simulink model "Clutchless_P2_Parallel_ETE"  (R2017b)
settings: Solver=FixedStepAuto  StartTime=0.0  StopTime=length(Speed)  FixedStep=0.01  MaxStep=0.01  RelTol=1e-3  EnableMultiTasking=on
PostLoadFcn:
  | , if any(exist('dsrtsu_mdlpostloadfcn', 'file') == [2, 3, 6]), try dsrtsu_mdlpostloadfcn('Execute', bdroot); catch fprintf('Error in PostLoadFcn (dsrtsu_mdlpostloadfcn) for model "%s":\n %s\n', bdroot, lasterr); end, end,
undefined symbols (not defined in the file): ABSEnable, Actuators, air, APP1_OOR, APP2_OOR, APP_Mismatch, Brk_Flt, cal, ClutchEngag, Clutchless_HSC_ETE, CS_On_Control, Driver, eng, Engine, EngOverTemp, ENGTRQ_MSMCH_Degraded_CP, ENGTRQ_MSMCH_ErrCritical_CP, ENGTRQ_MSMCH_LimpHome_CP, EngTrqMismatch, env, ess, ESSOverTemp, gb, KeyPos_Flt, KeyPosition, lib_Actuators, lib_Clutchless_HSC_ETE, lib_Driver, lib_EMachine_2017a, lib_Sensors_2017a, LossCAN, Machine, max_vehicle_rad_air_flow, MCUOverTemp, mot, MotDirMismatch, MotOverTemp, MotTrqMismatch, mph2ms, PRNDL_Flt, RegenBrkDisable, RegenFault, Sensors, ShiftLeverPosition, Speed, SW_CS_ON, SW_Engine_ON, t_amb, time, tloop
libraries: simulink x97, Pneumatic_lib x11, nesl_utility x9, EC2_libraries x7, powerlib_meascontrol x2, CalculationGallon x1, lib_Chassis x1, lib_DCDC x1, lib_Differential x1, lib_HVESS x1, fl_lib x1, lib_OBC x1
(part 4 of 9)

== system Clutchless_P2_Parallel_ETE/Camaro Plant Model/E-Machine/IMG Plant2/Motor_Plant/Efficiency Calcs ==
  Speed_rpm : Inport
  Torq_cmd_Nm : Inport  Port=2
  Batt_volt : Inport  Port=3
  Abs1 : Abs
  Constant : Constant
  Constant1 : Constant  Value=0
  Current_consum : Product  Inputs=*/
  Efficiency Map : Lookup_n-D  BreakpointsForDimension1=mot.map.trqindex  BreakpointsForDimension2=mot.map.spdindex  Table=mot.map.eff  InternalRulePriority=Speed  RndMeth=Simplest  InputSameDT=on
  Electrical power motoring : Product  Inputs=*//
  Electrical power regen : Product  Inputs=***
  Gain : Gain  Gain=2*3.14/60
  Gain1 : Gain  Gain=-1
  MCU_eff : Constant  Value=0.97
  Mech_power : Product  Inputs=**
  MinMax : MinMax  Function=max  Inputs=2
  MinMax1 : MinMax  Function=max  Inputs=2
  Saturation : Saturate  UpperLimit=400  LowerLimit=-400
  Switch : Switch  Criteria=u2 > Threshold
  Switch1 : Switch  Criteria=u2 > Threshold  Threshold=100
  min_eff : Constant  Value=0.1
  Mot_current : Outport
  Mech_power_W : Outport  Port=2
  Elec_power_W : Outport  Port=3
  wires:
  Constant1/1 -> Switch1/3
  Switch/1 -> Switch1/1  "Elec_power_W"
  Gain1/1 -> Saturation/1  "Mot_current_A"
  Constant/1 -> MinMax1/2
  MinMax1/1 -> Current_consum/2
  Efficiency Map/1 -> MinMax/1
  Switch1/1 -> Current_consum/1, Elec_power_W/1  "Elec_power_W"
  min_eff/1 -> MinMax/2
  Electrical power motoring/1 -> Switch/1
  MCU_eff/1 -> Electrical power motoring/3, Electrical power regen/3
  Mech_power/1 -> Mech_power_W/1, Electrical power regen/1, Electrical power motoring/1  "Mech_power_W"
  Abs1/1 -> Efficiency Map/1
  Batt_volt/1 -> MinMax1/1, Switch1/2
  Gain/1 -> Mech_power/1
  Saturation/1 -> Mot_current/1  "Mot_current_A"
  Current_consum/1 -> Gain1/1
  MinMax/1 -> Electrical power regen/2, Electrical power motoring/2
  Electrical power regen/1 -> Switch/3
  Torq_cmd_Nm/1 -> Switch/2, Abs1/1, Mech_power/2
  Speed_rpm/1 -> Gain/1, Efficiency Map/2

== system Clutchless_P2_Parallel_ETE/Camaro Plant Model/E-Machine/IMG Plant2/Thermal/Motor Thermal ==
  In1 : Inport
  Add1 : Sum  Inputs=+-
  Add2 : Sum
  Divide : Product  Inputs=*/
  Lower Limit : Subsystem  mask{Lolimit=t_amb+20}
      mask prompts: Lolimit "Lower Limit"
  Memory1 : Memory
  Motor Mass : Constant  Value=mot.plant.init.motor_mass
  Product : Product  RndMeth=Zero
  "Pump " : Constant  Value=0
  Specific Heat Cap Aluminum : Constant  Value=mot.plant.init.specific_heat
  tloop : Gain  Gain=tloop
  Out1 : Outport
  wires:
  Add1/1 -> tloop/1
  In1/1 -> Add1/1
  "Pump "/1 -> Add1/2
  Motor Mass/1 -> Product/1  "kg"
  tloop/1 -> Divide/1  "J"
  Divide/1 -> Add2/1
  Lower Limit/1(Out1) -> Memory1/1, Out1/1
  Add2/1 -> Lower Limit/1(In1)
  Memory1/1 -> Add2/2
  Product/1 -> Divide/2
  Specific Heat Cap Aluminum/1 -> Product/2  "J/kg*K"

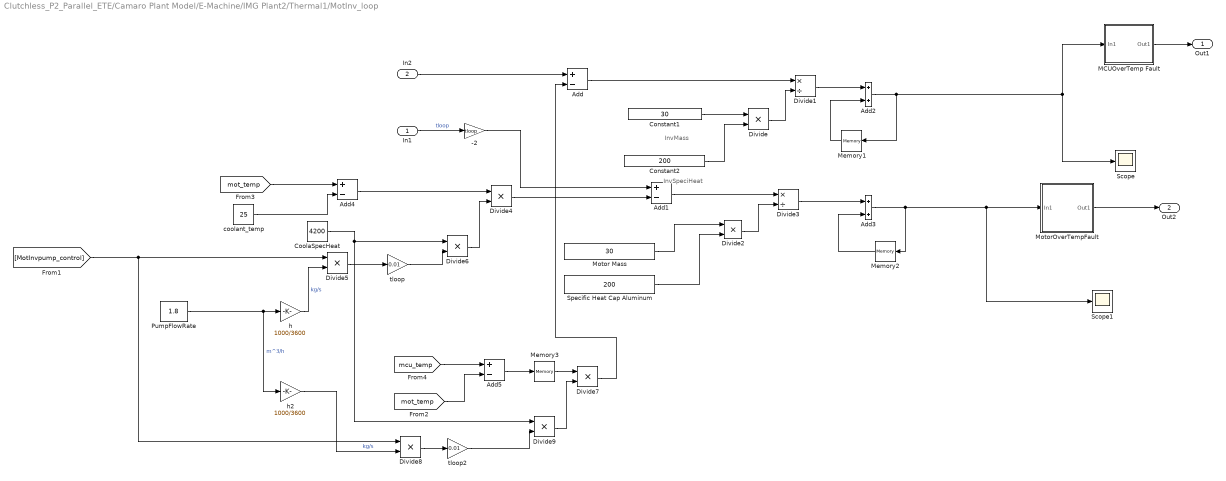
== system Clutchless_P2_Parallel_ETE/Camaro Plant Model/E-Machine/IMG Plant2/Thermal1/MotInv_loop ==
  note: InvMass
  note: InvSpeciHeat
  In1 : Inport
  In2 : Inport  Port=2
  -2 : Gain  Gain=tloop
  Add{,1,4..5} (4 alike) : Sum  Inputs=+-
  Add2 : Sum
  Add3 : Sum
  Constant1 : Constant  Value=30
  Constant2 : Constant  Value=200
  CoolaSpecHeat : Constant  Value=4200
  Divide{,2,4..9} (8 alike) : Product  Inputs=**
  Divide1 : Product  Inputs=*/
  Divide3 : Product  Inputs=*/
  MCUOverTemp Fault : Subsystem
  Memory1 : Memory  InitialCondition=25
  Memory2 : Memory  InitialCondition=25
  Memory3 : Memory
  Motor Mass : Constant  Value=30
  MotorOverTempFault : Subsystem
  PumpFlowRate : Constant  Value=1.8
  Scope : Scope
  Scope1 : Scope
  Specific Heat Cap Aluminum : Constant  Value=200
  coolant_temp : Constant  Value=25
  h : Gain  Gain=1000/3600
  h2 : Gain  Gain=1000/3600
  tloop : Gain  Gain=0.01
  tloop2 : Gain  Gain=0.01
  Out1 : Outport
  Out2 : Outport  Port=2
  wires:
  [MotInvpump_control] -> Divide5/1, Divide8/1
  -2/1 -> Add1/1
  In2/1 -> Add/1
  In1/1 -> -2/1  "tloop"
  [mot_temp] -> Add5/2
  [mcu_temp] -> Add5/1
  [mot_temp] -> Add4/1
  MotorOverTempFault/1(Out1) -> Out2/1
  MCUOverTemp Fault/1(Out1) -> Out1/1
  Memory3/1 -> Divide7/1
  Add5/1 -> Memory3/1
  Divide4/1 -> Add1/2
  tloop2/1 -> Divide9/2
  Divide8/1 -> tloop2/1
  Divide9/1 -> Divide7/2
  h2/1 -> Divide8/2  "kg/s"
  PumpFlowRate/1 -> h/1, h2/1  "m^3/h"
  CoolaSpecHeat/1 -> Divide9/1, Divide6/1
  tloop/1 -> Divide6/2
  h/1 -> Divide5/2  "kg/s"
  Divide7/1 -> Add/2
  Divide1/1 -> Add2/1
  Motor Mass/1 -> Divide2/1
  Constant2/1 -> Divide/2
  Divide2/1 -> Divide3/2
  Add2/1 -> Memory1/1, Scope/1, MCUOverTemp Fault/1(In1)
  Divide5/1 -> tloop/1
  Divide3/1 -> Add3/1
  Divide6/1 -> Divide4/2
  Add3/1 -> Memory2/1, MotorOverTempFault/1(In1), Scope1/1
  Add4/1 -> Divide4/1
  Memory2/1 -> Add3/2
  Add/1 -> Divide1/1
  Constant1/1 -> Divide/1
  Specific Heat Cap Aluminum/1 -> Divide2/2
  Divide/1 -> Divide1/2
  coolant_temp/1 -> Add4/2
  Memory1/1 -> Add2/2
  Add1/1 -> Divide3/1

== system Clutchless_P2_Parallel_ETE/Camaro Plant Model/E-Machine/IMG Plant2/Thermal1/Motor Thermal ==
  In1 : Inport
  Add1 : Sum  Inputs=+-
  Add2 : Sum
  Divide : Product  Inputs=*/
  Lower Limit : Subsystem  mask{Lolimit=t_amb+20}
      mask prompts: Lolimit "Lower Limit"
  Memory1 : Memory
  Motor Mass : Constant  Value=mot.plant.init.motor_mass
  Product : Product  RndMeth=Zero
  "Pump " : Constant  Value=0
  Specific Heat Cap Aluminum : Constant  Value=mot.plant.init.specific_heat
  tloop : Gain  Gain=tloop
  Out1 : Outport
  wires:
  Add1/1 -> tloop/1
  In1/1 -> Add1/1
  "Pump "/1 -> Add1/2
  Motor Mass/1 -> Product/1  "kg"
  tloop/1 -> Divide/1  "J"
  Divide/1 -> Add2/1
  Lower Limit/1(Out1) -> Memory1/1, Out1/1
  Add2/1 -> Lower Limit/1(In1)
  Memory1/1 -> Add2/2
  Product/1 -> Divide/2
  Specific Heat Cap Aluminum/1 -> Product/2  "J/kg*K"

== system Clutchless_P2_Parallel_ETE/Camaro Plant Model/E-Machine/IMG Plant2/Torque Calculation/electric machine filter ==
  trq : Inport
  Interval Test : simulink/Logic and Bit Operations/Interval Test  IntervalClosedRight=on  uplimit=0.5  IntervalClosedLeft=on  lowlimit=-0.5  OutDataTypeStr=boolean
  Switch : Switch  Threshold=0.5
  electric machine time response : TransferFcn  Denominator=[mot.plant.init.time_response 1]
  filtered : Outport
  wires:
  Switch/1 -> filtered/1
  trq/1 -> Switch/1, electric machine time response/1, Interval Test/1
  Interval Test/1 -> Switch/2
  electric machine time response/1 -> Switch/3

== system Clutchless_P2_Parallel_ETE/Camaro Plant Model/E-Machine/IMG Plant2/Torque Calculation/max torque  ==
  cmd : Inport
  speed : Inport  Port=2
  Memory : Memory
  Peak trq max - Motoring : Lookup  InputValues=mot.plant.init.regen.trq_max.idx1_spd  Table=mot.plant.init.motor.trq_max.map  LookUpMeth=Interpolation-Use End Values  SaturateOnIntegerOverflow=on
  Peak trq max - Regen : Lookup  InputValues=mot.plant.init.regen.trq_max.idx1_spd  Table=mot.plant.init.regen.trq_max.map  LookUpMeth=Interpolation-Use End Values  SaturateOnIntegerOverflow=on
  Switch1 : Switch  SaturateOnIntegerOverflow=on
  rad/s  to RPM : Gain  Gain=30/pi
  max torque : Outport
  wires:
  Peak trq max - Regen/1 -> Switch1/3
  rad/s  to RPM/1 -> Memory/1
  Memory/1 -> Peak trq max - Regen/1, Peak trq max - Motoring/1
  Switch1/1 -> max torque/1
  cmd/1 -> Switch1/2
  speed/1 -> rad/s  to RPM/1
  Peak trq max - Motoring/1 -> Switch1/1

== system Clutchless_P2_Parallel_ETE/Camaro Plant Model/E-Machine/Soft MCU/Subsystem/MCU_RollingAliveCnt ==
  Counter Free-Running : simulink/Sources/Counter Free-Running  NumBits=4  tsamp=-1
  Out1 : Outport
  wires:
  Counter Free-Running/1 -> Out1/1  "MCURollingAliveCnt [0 1 2 3]"

== system Clutchless_P2_Parallel_ETE/Camaro Plant Model/E-Machine/Soft MCU/Torque Calculation1/max torque  ==
  Req : Inport
  speed : Inport  Port=2
  torque : Inport  Port=3
  2-D Lookup Table : Lookup_n-D  Commented=on  BreakpointsForDimension1=mot.plant.init.eff_trq.idx2_trq  BreakpointsForDimension2=mot.plant.init.eff_trq.idx1_spd  Table=mot.plant.init.eff_trq.map  InternalRulePriority=Speed  RndMeth=Simplest  InputSameDT=on
  Abs : Abs  SaturateOnIntegerOverflow=on
  Abs1 : Abs  Commented=on
  Abs2 : Abs  Commented=on
  Constant : Constant  Commented=on  Value=84500
  Cont trq max - Motoring : Lookup  InputValues=mot.plant.init.motor.trq_cont.idx1_spd  Table=mot.plant.init.motor.trq_cont.map  LookUpMeth=Interpolation-Use End Values  SaturateOnIntegerOverflow=on
  Cont trq max - Regen : Lookup  InputValues=mot.plant.init.regen.trq_cont.idx1_spd  Table=mot.plant.init.regen.trq_cont.map  LookUpMeth=Interpolation-Use End Values  SaturateOnIntegerOverflow=on
  Divide : Product  Commented=on  Inputs=**/
  Divide by zero : Subsystem  Commented=on
  Gain2 : Gain  Commented=on  Gain=1/100
  Heat index : Subsystem
  Memory : Memory
  Peak trq max - Motoring : Lookup  Commented=on  InputValues=mot.plant.init.regen.trq_max.idx1_spd  Table=mot.plant.init.motor.trq_max.map  LookUpMeth=Interpolation-Use End Values  SaturateOnIntegerOverflow=on
  Peak trq max - Motoring1 : Lookup  InputValues=mot.plant.init.regen.trq_max.idx1_spd  Table=mot.plant.init.motor.trq_max.map  LookUpMeth=Interpolation-Use End Values  SaturateOnIntegerOverflow=on
  Peak trq max - Regen : Lookup  InputValues=mot.plant.init.regen.trq_max.idx1_spd  Table=mot.plant.init.regen.trq_max.map  LookUpMeth=Interpolation-Use End Values  SaturateOnIntegerOverflow=on
  Product2 : Product  SaturateOnIntegerOverflow=on  InputSameDT=on  OutDataTypeStr=Inherit: Same as first input
  Product3 : Product  SaturateOnIntegerOverflow=on  InputSameDT=on  OutDataTypeStr=Inherit: Same as first input
  Product5 : Product  SaturateOnIntegerOverflow=on  InputSameDT=on  OutDataTypeStr=Inherit: Same as first input
  RPM to rad/s : Gain  Commented=on  Gain=pi/30
  Sign : Signum
  Sum : Sum  SaturateOnIntegerOverflow=on  InputSameDT=on  OutDataTypeStr=Inherit: Same as first input
  Sum1 : Sum  Inputs=-+  SaturateOnIntegerOverflow=on  InputSameDT=on  OutDataTypeStr=Inherit: Same as first input
  Switch : Switch  SaturateOnIntegerOverflow=on
  Switch1 : Switch  SaturateOnIntegerOverflow=on
  cst : Constant
  max torque : Outport
  wires:
  Heat index/1(Heat index) -> Product2/2, Sum1/1
  cst/1 -> Sum1/2
  Product3/1 -> Sum/2
  Sum1/1 -> Product3/1
  Product2/1 -> Sum/1
  Switch1/1 -> Product3/2
  Switch/1 -> Heat index/1(cont torque), Product2/1
  Peak trq max - Regen/1 -> Switch1/3
  Cont trq max - Regen/1 -> Switch/3
  Cont trq max - Motoring/1 -> Switch/1
  torque/1 -> Heat index/2(torque)
  Abs/1 -> Product5/2
  Sum/1 -> Abs/1, Sign/1
  Product5/1 -> max torque/1
  Sign/1 -> Product5/1
  Memory/1 -> Cont trq max - Motoring/1, Cont trq max - Regen/1, Peak trq max - Motoring1/1, Peak trq max - Regen/1
  speed/1 -> Memory/1
  Constant/1 -> Divide/1
  RPM to rad/s/1 -> Divide by zero/1(In1)
  Abs2/1 -> 2-D Lookup Table/2
  Abs1/1 -> 2-D Lookup Table/1
  2-D Lookup Table/1 -> Gain2/1
  Gain2/1 -> Divide/2
  Req/1 -> Switch/2, Switch1/2
  Divide by zero/1(Out1) -> Divide/3
  Peak trq max - Motoring1/1 -> Switch1/1

== system Clutchless_P2_Parallel_ETE/Camaro Plant Model/E-Machine/Soft MCU/Torque Calculation2/max torque  ==
  Req : Inport
  speed : Inport  Port=2
  torque : Inport  Port=3
  2-D Lookup Table : Lookup_n-D  Commented=on  BreakpointsForDimension1=mot.plant.init.eff_trq.idx2_trq  BreakpointsForDimension2=mot.plant.init.eff_trq.idx1_spd  Table=mot.plant.init.eff_trq.map  InternalRulePriority=Speed  RndMeth=Simplest  InputSameDT=on
  Abs : Abs  SaturateOnIntegerOverflow=on
  Abs1 : Abs  Commented=on
  Abs2 : Abs  Commented=on
  Constant : Constant  Commented=on  Value=84500
  Cont trq max - Motoring : Lookup  InputValues=mot.plant.init.motor.trq_cont.idx1_spd  Table=mot.plant.init.motor.trq_cont.map  LookUpMeth=Interpolation-Use End Values  SaturateOnIntegerOverflow=on
  Cont trq max - Regen : Lookup  InputValues=mot.plant.init.regen.trq_cont.idx1_spd  Table=mot.plant.init.regen.trq_cont.map  LookUpMeth=Interpolation-Use End Values  SaturateOnIntegerOverflow=on
  Divide : Product  Commented=on  Inputs=**/
  Divide by zero : Subsystem  Commented=on
  Gain2 : Gain  Commented=on  Gain=1/100
  Heat index : Subsystem
  Memory : Memory
  Peak trq max - Motoring : Lookup  Commented=on  InputValues=mot.plant.init.regen.trq_max.idx1_spd  Table=mot.plant.init.motor.trq_max.map  LookUpMeth=Interpolation-Use End Values  SaturateOnIntegerOverflow=on
  Peak trq max - Motoring1 : Lookup  InputValues=mot.plant.init.regen.trq_max.idx1_spd  Table=mot.plant.init.motor.trq_max.map  LookUpMeth=Interpolation-Use End Values  SaturateOnIntegerOverflow=on
  Peak trq max - Regen : Lookup  InputValues=mot.plant.init.regen.trq_max.idx1_spd  Table=mot.plant.init.regen.trq_max.map  LookUpMeth=Interpolation-Use End Values  SaturateOnIntegerOverflow=on
  Product2 : Product  SaturateOnIntegerOverflow=on  InputSameDT=on  OutDataTypeStr=Inherit: Same as first input
  Product3 : Product  SaturateOnIntegerOverflow=on  InputSameDT=on  OutDataTypeStr=Inherit: Same as first input
  Product5 : Product  SaturateOnIntegerOverflow=on  InputSameDT=on  OutDataTypeStr=Inherit: Same as first input
  RPM to rad/s : Gain  Commented=on  Gain=pi/30
  Sign : Signum
  Sum : Sum  SaturateOnIntegerOverflow=on  InputSameDT=on  OutDataTypeStr=Inherit: Same as first input
  Sum1 : Sum  Inputs=-+  SaturateOnIntegerOverflow=on  InputSameDT=on  OutDataTypeStr=Inherit: Same as first input
  Switch : Switch  SaturateOnIntegerOverflow=on
  Switch1 : Switch  SaturateOnIntegerOverflow=on
  cst : Constant
  max torque : Outport
  wires:
  Heat index/1(Heat index) -> Product2/2, Sum1/1
  cst/1 -> Sum1/2
  Product3/1 -> Sum/2
  Sum1/1 -> Product3/1
  Product2/1 -> Sum/1
  Switch1/1 -> Product3/2
  Switch/1 -> Heat index/1(cont torque), Product2/1
  Peak trq max - Regen/1 -> Switch1/3
  Cont trq max - Regen/1 -> Switch/3
  Cont trq max - Motoring/1 -> Switch/1
  torque/1 -> Heat index/2(torque)
  Abs/1 -> Product5/2
  Sum/1 -> Abs/1, Sign/1
  Product5/1 -> max torque/1
  Sign/1 -> Product5/1
  Memory/1 -> Cont trq max - Motoring/1, Cont trq max - Regen/1, Peak trq max - Motoring1/1, Peak trq max - Regen/1
  speed/1 -> Memory/1
  Constant/1 -> Divide/1
  RPM to rad/s/1 -> Divide by zero/1(In1)
  Abs2/1 -> 2-D Lookup Table/2
  Abs1/1 -> 2-D Lookup Table/1
  2-D Lookup Table/1 -> Gain2/1
  Gain2/1 -> Divide/2
  Req/1 -> Switch/2, Switch1/2
  Divide by zero/1(Out1) -> Divide/3
  Peak trq max - Motoring1/1 -> Switch1/1

== system Clutchless_P2_Parallel_ETE/Camaro Plant Model/ICE Simple1/Engine Plant Modified/Core Engine/Core Engine1 ==
  Engine Speed (RPM) : Inport
  CO : Lookup2D  RowIndex=Engine.Engine.Emissions.SPEED  ColumnIndex=Engine.Engine.Emissions.TQ  Table=Engine.Engine.Emissions.CO/1000  LookUpMeth=Interpolation-Use End Values
  CO2 : Lookup2D  RowIndex=Engine.Engine.Emissions.SPEED  ColumnIndex=Engine.Engine.Emissions.TQ  Table=Engine.Engine.Emissions.CO2/1000  LookUpMeth=Interpolation-Use End Values
  Controlled Pneumatic Flow Rate Source : Pneumatic_lib/Pneumatic Sources/Controlled Pneumatic Flow Rate Source
  Fuel Flow : Lookup2D  RowIndex=Engine.Engine.FuelFlow.SPEED  ColumnIndex=Engine.Engine.FuelFlow.TQ  Table=Engine.Engine.FuelFlow.FuelFlow  LookUpMeth=Interpolation-Use End Values
  HC : Lookup2D  RowIndex=Engine.Engine.Emissions.SPEED  ColumnIndex=Engine.Engine.Emissions.TQ  Table=Engine.Engine.Emissions.HC/1000  LookUpMeth=Interpolation-Use End Values
  Half of Displacement : Gain  Gain=Engine.DisplacedVolume/(2*1000)
  Ideal Gas Constant R : Gain  Gain=287
  Kg/s to g/s : Gain  Gain=1000
  LP Filter1 : TransferFcn  Denominator=[0.001 1]
  Memory : Memory
  NOx : Lookup2D  RowIndex=Engine.Engine.Emissions.SPEED  ColumnIndex=Engine.Engine.Emissions.TQ  Table=Engine.Engine.Emissions.NOx/1000  LookUpMeth=Interpolation-Use End Values
  Power Enrichment Torque Boundary vs Speed : Lookup_n-D  NumberOfTableDimensions=1  BreakpointsForDimension1=Engine.Engine.PEBound.SPEED  Table=Engine.Engine.PEBound.PEBound  ExtrapMethod=Clip  InternalRulePriority=Speed  RndMeth=Simplest  InputSameDT=on
  Product : Product  Inputs=***
  RPM to RPS : Gain  Gain=1/60
  Relational Operator : RelationalOperator  Operator=>  OutDataTypeStr=boolean  RndMeth=Nearest
  Simulink-PS Converter2 : nesl_utility/Simulink-PS Converter  PhysicalDomain=network_engine_domain  SubClassName=ps_input  LeftPortType=input  RightPortType=output  PseudoPeriodic=off  Frequencies=[]  NoiseDistribution=none  NoiseParameters=[]  Unit=kg/s  AffineConversion=off  FilteringAndDerivatives=zero  SimscapeFilterOrder=1  InputFilterTimeConstant=.001  UdotUserProvided=0
  Speed-Density Mass Flow : Product  Inputs=*/
  Torque : Lookup2D  RowIndex=Engine.Engine.TQ.SPEED  ColumnIndex=Engine.Engine.TQ.MAF  Table=Engine.Engine.TQ.TQ  LookUpMeth=Interpolation-Use End Values
  Upstream States : Subsystem
  Volumetric Efficiency : Lookup2D  RowIndex=Engine.Engine.VE.MAP  ColumnIndex=Engine.Engine.VE.SPEED  Table=Engine.Engine.VE.VE  LookUpMeth=Interpolation-Use End Values
  A : PMIOPort  Port=1  Side=Left
  B : PMIOPort  Port=2  Side=Right
  Brake Torque (Nm) : Outport
  Fuel Flow (g/s) : Outport  Port=2
  PE Status : Outport  Port=3
  HC (g/s) : Outport  Port=4
  CO (g/s) : Outport  Port=5
  NOx (g/s) : Outport  Port=6
  CO2 (g/s) : Outport  Port=7
  Intake Port Airflow (g/s) : Outport  Port=8
  wires:
  Upstream States/1(P (Pa)) -> Volumetric Efficiency/1, Product/3
  Volumetric Efficiency/1 -> Product/1
  Ideal Gas Constant R/1 -> Speed-Density Mass Flow/2
  Product/1 -> Speed-Density Mass Flow/1
  Upstream States/2(T (K)) -> Ideal Gas Constant R/1
  RPM to RPS/1 -> Half of Displacement/1
  Half of Displacement/1 -> Product/2
  Kg/s to g/s/1 -> [INTAKEPORTFLOW]
  Torque/1 -> Brake Torque (Nm)/1, Relational Operator/1, Memory/1  "Brake Torque"
  [INTAKEPORTFLOW] -> Torque/2
  Fuel Flow/1 -> Fuel Flow (g/s)/1  "Fuel Flow"
  Engine Speed (RPM)/1 -> Torque/1, Fuel Flow/1, HC/1, CO/1, NOx/1, Power Enrichment Torque Boundary vs Speed/1, CO2/1, Volumetric Efficiency/2, RPM to RPS/1
  Memory/1 -> CO2/2, NOx/2, CO/2, HC/2, Fuel Flow/2
  Power Enrichment Torque Boundary vs Speed/1 -> Relational Operator/2
  Relational Operator/1 -> PE Status/1
  HC/1 -> HC (g/s)/1
  CO/1 -> CO (g/s)/1
  NOx/1 -> NOx (g/s)/1
  CO2/1 -> CO2 (g/s)/1
  [INTAKEPORTFLOW] -> Intake Port Airflow (g/s)/1
  Speed-Density Mass Flow/1 -> LP Filter1/1, Kg/s to g/s/1
  LP Filter1/1 -> Simulink-PS Converter2/1
  connections:
  A/RConn1 -- Controlled Pneumatic Flow Rate Source/RConn1 -- Upstream States/LConn1
  Simulink-PS Converter2/RConn1 -- Controlled Pneumatic Flow Rate Source/RConn2
  B/RConn1 -- Controlled Pneumatic Flow Rate Source/LConn1

== system Clutchless_P2_Parallel_ETE/Camaro Plant Model/ICE Simple1/Engine Plant Modified/Core Engine/Crank Process/function ==
  EngSpd : Inport
  f : TriggerPort  TriggerType=function-call  VariantControl=Variant
      settings: CopyFcn=Stateflow.SLINSF.SimulinkMan.removeBlockPreDeleteFcn  PreDeleteFcn=Stateflow.SLINSF.SimulinkMan.unsafePredeleteFcn
  1-D Lookup Table : Lookup_n-D  NumberOfTableDimensions=1  BreakpointsForDimension1=[0 50 120 210 300 320 340 350 400]  Table="[90 90 90 10 5 5  5 5 5]"  InternalRulePriority=Speed  RndMeth=Simplest  InputSameDT=on
  CrankTrq : Outport
  wires:
  EngSpd/1 -> 1-D Lookup Table/1
  1-D Lookup Table/1 -> CrankTrq/1

== system Clutchless_P2_Parallel_ETE/Camaro Plant Model/ICE Simple1/Engine Plant Modified/Core Engine/EngEfficiency1 ==
  note: Mechanical Power [W]
  Torque : Inport
  Speed : Inport  Port=2
  Fuel Consumption : Inport  Port=3
  Divide by Zero Fix : Subsystem
  Divide_by_Zero_Fix1 : EC2_libraries/Divide_by_Zero_Fix  Commented=on
  From1 : From  Commented=on  GotoTag=Wh_out
  From2 : From  Commented=on  GotoTag=Wh_in
  Goto1 : Goto  Commented=on  GotoTag=Wh_out
  Goto2 : Goto  Commented=on  GotoTag=Wh_in
  Integrator1 : Integrator  Commented=on  LimitOutput=on  LowerSaturationLimit=0
  Integrator2 : Integrator  Commented=on  LimitOutput=on  LowerSaturationLimit=0
  OnlyPositiveEnergy : Saturate  Commented=on  UpperLimit=inf  LowerLimit=0
  Percentage Efficiency : Gain  Gain=100
  Product : Product  RndMeth=Zero
  "RPM to rad/s " : Gain  Gain=pi/30
  Scope : Scope  NumInputPorts=2
  Specific Energy LHV in J/kg : Gain  Gain=Engine.Fuel.Lower_Heating_Value/1000
  Sum : Sum  Inputs=-+
  To Workspace7 : ToWorkspace  Commented=on  VariableName=eng_Wh_pos_eff_hist  SampleTime=-1
      settings: Decimation=WORKSPACE_DECIMATION
  engine_efficiency : Scope
  limit_efficiency[0-100%] : Saturate  UpperLimit=100  LowerLimit=0
  PowerLoss : Outport
  wires:
  limit_efficiency[0-100%]/1 -> engine_efficiency/1
  Sum/1 -> PowerLoss/1  "Losses [W]"
  Fuel Consumption/1 -> Specific Energy LHV in J/kg/1
  Specific Energy LHV in J/kg/1 -> Divide by Zero Fix/2(Divide), Sum/2, Integrator2/1, Scope/2  "Thermal Power [W]"
  Torque/1 -> Product/2  "Nm"
  Speed/1 -> "RPM to rad/s "/1  "rpm"
  Percentage Efficiency/1 -> limit_efficiency[0-100%]/1  "Efficiency [%]"
  Divide by Zero Fix/1(Output) -> Percentage Efficiency/1
  Product/1 -> Scope/1, Divide by Zero Fix/1(Multiply), OnlyPositiveEnergy/1, Sum/1  "wer [W]"
  Divide_by_Zero_Fix1/1 -> To Workspace7/1
  From1/1 -> Divide_by_Zero_Fix1/1
  From2/1 -> Divide_by_Zero_Fix1/2
  Integrator1/1 -> Goto1/1
  OnlyPositiveEnergy/1 -> Integrator1/1
  Integrator2/1 -> Goto2/1
  "RPM to rad/s "/1 -> Product/1

== system Clutchless_P2_Parallel_ETE/Camaro Plant Model/ICE Simple1/Engine Plant Modified/Core Engine/EngineThermal1 ==
  note: Temp Delta C deg
  PowerLoss : Inport
  Divide : Product  Inputs=*/
  Divide1 : Product  Inputs=**
  Engine Mass : Constant  Value=Engine.Mass
  Memory : Memory  InitialCondition=Engine.Init_T_amb
  Memory1 : Memory
  Product : Product  RndMeth=Zero
  Specific Heat Cap Aluminum : Constant  Value=Engine.Specific_Heat
  Sum : Sum  Inputs=|++
  Sum1 : Sum  Inputs=|+-
  Terminator : Terminator
  tloop : Constant  Value=0.01
  Temp[degC] : Outport
  tag scope: Heat_Transfer_Eng=global
  wires:
  Memory1/1 -> Sum1/2
  Divide1/1 -> Divide/1  "J"
  Sum1/1 -> Divide1/2
  Memory/1 -> Sum/2
  PowerLoss/1 -> Sum1/1, [Heat_Transfer_Eng]  "J/s"
  Engine Mass/1 -> Product/1  "kg"
  Specific Heat Cap Aluminum/1 -> Product/2  "J/kg*K"
  Product/1 -> Divide/2
  Sum/1 -> Memory/1, Temp[degC]/1
  Divide/1 -> Sum/1
  tloop/1 -> Divide1/1
  [Heat_Reject_Eng] -> Memory1/1
  [Heat_Transfer_Eng] -> Terminator/1

== system Clutchless_P2_Parallel_ETE/Camaro Plant Model/ICE Simple1/Engine Plant Modified/Core Engine/Intake Manifold1 ==
  Heat-Transfer Neglected : fl_lib/Thermal/Thermal Elements/Perfect Insulator  T_specify=off  T_priority=None  T=0 K  T_nominal_specify=off  T_nominal_unit=K  T_nominal_value=1
      settings: SourceProductName=Simscape
  Intake Manifold Volume1 : Pneumatic_lib/Pneumatic Elements/Constant Volume Pneumatic Chamber  Volume=Engine.IntakeManifold.Volume l  pressure_specify=on  pressure_priority=High  pressure=26 kPa  pressure_nominal_specify=off  pressure_nominal_unit=Pa  pressure_nominal_value=1  temperature_specify=on  temperature_priority=High  temperature=20 K  temperature_nominal_specify=off  temperature_nominal_unit=K  temperature_nominal_value=1  gas_flow_specify=off  gas_flow_priority=High  gas_flow=0 kg/s  gas_flow_nominal_specify=off  gas_flow_nominal_unit=kg/s  gas_flow_nominal_value=1  heat_flow_specify=off  heat_flow_priority=High  heat_flow=0 J/s  heat_flow_nominal_specify=off  heat_flow_nominal_unit=J/s  heat_flow_nominal_value=1  heat_exch_flow_specify=off  heat_exch_flow_priority=High  heat_exch_flow=0 J/s  heat_exch_flow_nominal_specify=off  heat_exch_flow_nominal_unit=J/s  heat_exch_flow_nominal_value=1
  Node Potential Sensor : Subsystem
  A : PMIOPort  Port=1  Side=Left
  MAP : Outport
  MAT : Outport  Port=2
  wires:
  Node Potential Sensor/1(P (KPa)) -> MAP/1
  Node Potential Sensor/2(T (C)) -> MAT/1
  connections:
  Node Potential Sensor/LConn1 -- Intake Manifold Volume1/LConn1 -- A/RConn1
  Intake Manifold Volume1/LConn2 -- Heat-Transfer Neglected/LConn1

== system Clutchless_P2_Parallel_ETE/Camaro Plant Model/ICE Simple1/Engine Plant Modified/Core Engine/Throttle Body1 ==
  Throttle Position % CMD : Inport
  CA vs TP : Lookup  InputValues=Engine.Throttle.CA.TPP  Table=Engine.Throttle.CA.CA  LookUpMeth=Interpolation-Use End Values
  ETC Actuator Dynamics : TransferFcn  Denominator=[0.04 1]
  PS-Simulink Converter : nesl_utility/PS-Simulink Converter  PhysicalDomain=network_engine_domain  SubClassName=ps_output  LeftPortType=input  RightPortType=output  PseudoPeriodic=off  Frequencies=[]  Unit=g/s  AffineConversion=off
  PS-Simulink Converter1 : nesl_utility/PS-Simulink Converter  PhysicalDomain=network_engine_domain  SubClassName=ps_output  LeftPortType=input  RightPortType=output  PseudoPeriodic=off  Frequencies=[]  Unit=J/s  AffineConversion=off
  Pneumatic Mass & Heat Flow Sensor : Pneumatic_lib/Pneumatic Sensors/Pneumatic Mass & Heat Flow Sensor
  Simulink-PS Converter : nesl_utility/Simulink-PS Converter  PhysicalDomain=network_engine_domain  SubClassName=ps_input  LeftPortType=input  RightPortType=output  PseudoPeriodic=off  Frequencies=[]  NoiseDistribution=none  NoiseParameters=[]  Unit=m^2  AffineConversion=off  FilteringAndDerivatives=zero  SimscapeFilterOrder=1  InputFilterTimeConstant=.001  UdotUserProvided=0
  Terminator : Terminator
  Throttle Throat : Pneumatic_lib/Pneumatic Elements/Variable Area Pneumatic Orifice  Cd=1  Area0=1e-7 m^2  G_specify=off  G_priority=High  G=0 kg/s  G_nominal_specify=off  G_nominal_unit=kg/s  G_nominal_value=1  Q1_specify=off  Q1_priority=High  Q1=0 J/s  Q1_nominal_specify=off  Q1_nominal_unit=J/s  Q1_nominal_value=1  Q2_specify=off  Q2_priority=High  Q2=0 J/s  Q2_nominal_specify=off  Q2_nominal_unit=J/s  Q2_nominal_value=1  p1_specify=off  p1_priority=High  p1=1e+5 Pa  p1_nominal_specify=off  p1_nominal_unit=Pa  p1_nominal_value=1  p2_specify=off  p2_priority=High  p2=1e+5 Pa  p2_nominal_specify=off  p2_nominal_unit=Pa  p2_nominal_value=1  T1_specify=off  T1_priority=High  T1=300 K  T1_nominal_specify=off  T1_nominal_unit=K  T1_nominal_value=1  T2_specify=off  T2_priority=High  T2=300 K  T2_nominal_specify=off  T2_nominal_unit=K  T2_nominal_value=1
  B : PMIOPort  Port=1  Side=Right
  A : PMIOPort  Port=2  Side=Left
  Throttle Flow kg/s : Outport
  Throttle Position % : Outport  Port=2
  wires:
  ETC Actuator Dynamics/1 -> Throttle Position %/1, CA vs TP/1
  CA vs TP/1 -> Simulink-PS Converter/1
  PS-Simulink Converter/1 -> Throttle Flow kg/s/1
  PS-Simulink Converter1/1 -> Terminator/1
  Throttle Position % CMD/1 -> ETC Actuator Dynamics/1
  connections:
  Simulink-PS Converter/RConn1 -- Throttle Throat/LConn2
  Throttle Throat/LConn1 -- A/RConn1
  Pneumatic Mass & Heat Flow Sensor/RConn2 -- PS-Simulink Converter/LConn1
  Pneumatic Mass & Heat Flow Sensor/RConn3 -- PS-Simulink Converter1/LConn1
  Throttle Throat/RConn1 -- Pneumatic Mass & Heat Flow Sensor/LConn1
  Pneumatic Mass & Heat Flow Sensor/RConn1 -- B/RConn1

== system Clutchless_P2_Parallel_ETE/Camaro Plant Model/ICE Simple1/Engine Plant Modified/Radiator/Divide by Zero Fix ==
  Multiply : Inport
  Divide : Inport  Port=2
  Compare To Zero : simulink/Logic and Bit Operations/Compare To Zero  relop===  OutDataTypeStr=boolean
  Constant1 : Constant  Value=0
  Constant2 : Constant
  Product2 : Product  Inputs=/*  SaturateOnIntegerOverflow=on  InputSameDT=on  OutDataTypeStr=Inherit: Same as first input
  Switch : Switch  Threshold=1
  Switch1 : Switch  Threshold=1
  Output : Outport
  wires:
  Multiply/1 -> Product2/2
  Switch1/1 -> Output/1
  Constant1/1 -> Switch1/1
  Product2/1 -> Switch1/3
  Switch/1 -> Product2/1
  Divide/1 -> Switch/3, Compare To Zero/1
  Constant2/1 -> Switch/1
  Compare To Zero/1 -> Switch1/2, Switch/2

== system Clutchless_P2_Parallel_ETE/Camaro Plant Model/ICE Simple1/Soft ECM/Fuel Consumption/Divide by Zero Fix ==
  Divide : Inport
  Multiply : Inport  Port=2
  Compare To Zero : simulink/Logic and Bit Operations/Compare To Zero  relop===  OutDataTypeStr=boolean
  Constant1 : Constant  Value=0
  Constant2 : Constant
  Divide1 : InportShadow
  Product2 : Product  Inputs=/*  SaturateOnIntegerOverflow=on  InputSameDT=on  OutDataTypeStr=Inherit: Same as first input
  Switch : Switch  Criteria=u2 > Threshold
  Switch1 : Switch  Criteria=u2 ~= 0
  Output : Outport
  wires:
  Multiply/1 -> Product2/2
  Switch1/1 -> Output/1
  Constant1/1 -> Switch1/3
  Product2/1 -> Switch1/1
  Switch/1 -> Product2/1
  Constant2/1 -> Switch/1
  Compare To Zero/1 -> Switch/2
  Divide/1 -> Switch/3, Compare To Zero/1
  Divide1/1 -> Switch1/2

== system Clutchless_P2_Parallel_ETE/Camaro Plant Model/ICE Simple1/Soft ECM/Fuel Consumption/Divide by Zero Fix1 ==
  Divide : Inport
  Multiply : Inport  Port=2
  Compare To Zero : simulink/Logic and Bit Operations/Compare To Zero  relop===  OutDataTypeStr=boolean
  Constant1 : Constant  Value=0
  Constant2 : Constant
  Divide1 : InportShadow
  Product2 : Product  Inputs=/*  SaturateOnIntegerOverflow=on  InputSameDT=on  OutDataTypeStr=Inherit: Same as first input
  Switch : Switch  Criteria=u2 > Threshold
  Switch1 : Switch  Criteria=u2 ~= 0
  Output : Outport
  wires:
  Divide1/1 -> Switch1/2
  Multiply/1 -> Product2/2
  Compare To Zero/1 -> Switch/2
  Constant1/1 -> Switch1/3
  Switch1/1 -> Output/1
  Switch/1 -> Product2/1
  Constant2/1 -> Switch/1
  Product2/1 -> Switch1/1
  Divide/1 -> Switch/3, Compare To Zero/1

== system Clutchless_P2_Parallel_ETE/Clutchless_HSC_ETE/HSC/Camaro Fault Detection/Component Diagnostic/Driver Input Diagnostic ==
  note: Driver_CompStatus
      | 1 = Component Online
      | 0 = Component Offline
  note: APP1
      | APP2
      | BPP
      | Driver Component Status
      |
      | 1
      | 1
      | 1
      | 1
      |
      | 0
      | 1
      | 1
      | 1
      |
      | 1
      | 0
      | 1
      | 1
      |
      | 0
      | 0
      | 1
      | 0
      |
      | 1
      | 1
      | 0
      | 0
      |
      | 0
      | 0
      | 0
      | 0
  In1 : Inport
  Bus Selector : BusSelector  OutputSignals=Driver_SigDiag.Drv_APP1_[%]_SigValid,Driver_SigDiag.Drv_APP2_[%]_SigValid,Driver_SigDiag.Drv_APP_Agree,Driver_SigDiag.Drv_BPP_[%]_SigValid,Driver_SigDiag.Drv_KeyPos_[0 3]_SigValid,Driver_SigDiag.Drv_PRNDL_SigValid,Driver_SigDiag.Brake_Failed
  Driver_Input_Diag : Stateflow chart  TreatAsAtomicUnit=on
  Logical Operator : Logic  Inputs=3  AllPortsSameDT=off  OutDataTypeStr=boolean
  Out1 : Outport
  wires:
  In1/1 -> Bus Selector/1
  Bus Selector/1 -> Logical Operator/1  "<Drv_APP1_[%]_SigValid>"
  Bus Selector/2 -> Logical Operator/2  "<Drv_APP2_[%]_SigValid>"
  Bus Selector/4 -> Driver_Input_Diag/2(Drv_BPP_SigValid)  "<Drv_BPP_[%]_SigValid>"
  Driver_Input_Diag/1(Driver_Input_Status) -> Out1/1  "Driver_Input_Status"
  Logical Operator/1 -> Driver_Input_Diag/1(APP_Valid)  "APP_Valid"
  Bus Selector/3 -> Logical Operator/3  "<Drv_APP_Agree>"
  Bus Selector/5 -> Driver_Input_Diag/3(KeyPos)  "<Drv_KeyPos_[0 3]_SigValid>"
  Bus Selector/6 -> Driver_Input_Diag/4(PRNDL)  "<Drv_PRNDL_SigValid>"
  Bus Selector/7 -> Driver_Input_Diag/5(BrakeFail)  "<Brake_Failed>"

== system Clutchless_P2_Parallel_ETE/Clutchless_HSC_ETE/HSC/Camaro Fault Detection/Component Diagnostic/ESS Component Diagnostic ==
  note: (Need modify)
  In1 : Inport
  BMS_CompDiag1 : Stateflow chart  TreatAsAtomicUnit=on
  Bus Selector : BusSelector  OutputSignals=ESS_SigDiag.BMS_RollingAliveActive_SigValid,ESS_SigDiag.BMS_contactorsFailed_Detected,ESS_SigDiag.BMS_essTemp_[degC]_SigValid,ESS_SigDiag.essTempRange[0_4],ESS_SigDiag.BMS_essSOC_0_1_SigValid,ESS_SigDiag.essTempRange[0_4],ESS_SigDiag.essCur_A_SigValid,ESS_SigDiag.BMSgdf_SigValid,Driver_SigDiag.Drv_KeyPos_[0 3]_SigValid
  Compare To Zero : simulink/Logic and Bit Operations/Compare To Zero  relop===  OutDataTypeStr=boolean
  Data Type Conversion : DataTypeConversion
  HVessFltReset : Constant
  Logical Operator : Logic  Operator=OR  AllPortsSameDT=off  OutDataTypeStr=boolean
  Logical Operator1 : Logic  AllPortsSameDT=off  OutDataTypeStr=boolean
  Terminator : Terminator
  Terminator1 : Terminator
  Out1 : Outport
  wires:
  In1/1 -> Bus Selector/1
  Bus Selector/1 -> BMS_CompDiag1/1(BMS_RollingAliveActive_SigValid)  "<BMS_RollingAliveActive_SigValid>"
  Bus Selector/2 -> [contactorsFailed_Detected], BMS_CompDiag1/2(BMS_contactorsFailed_SigValid)  "<BMS_contactorsFailed_Detected>"
  BMS_CompDiag1/1(BMS_Status) -> Out1/1  "BMS_Status"
  Bus Selector/4 -> Terminator/1  "<essTempRange[0_4]>"
  Bus Selector/3 -> Data Type Conversion/1  "<BMS_essTemp_[degC]_SigValid>"
  Data Type Conversion/1 -> BMS_CompDiag1/3(BMS_essTemp_SigValid)  "BMS_essTemp_SigValid"
  Bus Selector/5 -> BMS_CompDiag1/4(BMS_essSOC_0_1_SigValid)  "<BMS_essSOC_0_1_SigValid>"
  Bus Selector/6 -> Terminator1/1  "<essTempRange[0_4]>"
  Bus Selector/7 -> BMS_CompDiag1/5(essCur_A_SigValid)  "<essCur_A_SigValid>"
  Bus Selector/9 -> Compare To Zero/1  "<Drv_KeyPos_[0 3]_SigValid>"
  Compare To Zero/1 -> Logical Operator/1
  HVessFltReset/1 -> Logical Operator/2
  Logical Operator/1 -> BMS_CompDiag1/7(ClearFault)
  Bus Selector/8 -> Logical Operator1/2  "<BMSgdf_SigValid>"
  Logical Operator1/1 -> BMS_CompDiag1/6(ess_GroundFault)
  [contactorsFailed_Detected] -> Logical Operator1/1

== system Clutchless_P2_Parallel_ETE/Clutchless_HSC_ETE/HSC/Camaro Fault Detection/Component Diagnostic/Engine Component Diagnostic ==
  note: Eng_Torq_MsmchLevel
      | 1:Normal torque
      | 2: Limit max power
      | 3: Deliver creep torque
      | 4: offline
  note: ENGTRQ_MSMCH_Degraded_CP (40Nm): ENGTRQ_Degraded fault code.
      | ENGTRQ_MSMCH_LimpHome_CP (70Nm): ENGTRQ_LimpHome
      | ENGTRQ_MSMCH_ErrCritical_CP (100Nm): ENGTRQ_ErrCritical
  note: Eng_tempRange
      | 1: normal
      | 2: high range
      | 3:above max
  note: add the temperature, mismatch torquesignal and have different status to the component
  note: 0: component needs to be offline
      | 1: component needs torque plant to deliver creep torque
      | 2: component needs torque plant to limit maximum torque delivery
      | 3: component needs torque plant to operate normally
  note: Notes
  In1 : Inport
  Bus Selector : BusSelector  OutputSignals=Engine_SigDiag.ECMRollingAliveActive,Engine_SigDiag.engTrqCmdRecvd_SigValid,Engine_SigDiag.ECMTrqCmd_Nm,Engine_SigDiag.EngActStdyStTorq_Nm,Engine_SigDiag.EngRunAtValid,Engine_SigDiag.Engine_Speed_rpm_SigValid,Engine_SigDiag.Eng_TempValid,Engine_SigDiag.Eng_TempRange[123],Driver_SigDiag.Drv_KeyPos_[0 3]_SigValid
  Bus Selector1 : BusSelector  OutputSignals=Eng_Torque_Mismch_Critical
  Compare To Zero : simulink/Logic and Bit Operations/Compare To Zero  relop===  OutDataTypeStr=boolean
  ECM_CompDiag : Stateflow chart  TreatAsAtomicUnit=on
  Eng_FltReset : Constant
  Eng_Torq_MsmchLevel : Stateflow chart  Commented=on  TreatAsAtomicUnit=on
  Logical Operator : Logic  Operator=OR  AllPortsSameDT=off  OutDataTypeStr=boolean
  Override  engTrqCmd : Subsystem
  Terminator1 : Terminator
  TorqMismatch Detection : Subsystem
  Out1 : Outport
  Out2 : Outport  Port=2
  wires:
  In1/1 -> Bus Selector/1
  Bus Selector/1 -> ECM_CompDiag/1(ECM_RollingAliveActive)  "<ECMRollingAliveActive>"
  Bus Selector/2 -> Override  engTrqCmd/1(In1)  "<engTrqCmdRecvd_SigValid>"
  Bus Selector/6 -> ECM_CompDiag/4(Engine_Speed_rpm_SigValid)  "<Engine_Speed_rpm_SigValid>"
  ECM_CompDiag/1(ECM_Status) -> Out1/1  "ECM_Status"
  Compare To Zero/1 -> Logical Operator/1
  Eng_FltReset/1 -> Logical Operator/2
  Logical Operator/1 -> ECM_CompDiag/6(ClearFault)
  Bus Selector/9 -> Compare To Zero/1  "<Drv_KeyPos_[0 3]_SigValid>"
  Bus Selector/7 -> Terminator1/1  "<Eng_TempValid>"
  Bus Selector/8 -> ECM_CompDiag/5(Eng_TempRange_123)  "<Eng_TempRange[123]>"
  Bus Selector/3 -> TorqMismatch Detection/1(In1)  "<ECMTrqCmd_Nm>"
  Bus Selector/4 -> TorqMismatch Detection/2(In2)  "<EngActStdyStTorq_Nm>"
  Bus Selector/5 -> TorqMismatch Detection/3(In3)  "<EngRunAtValid>"
  TorqMismatch Detection/1(Eng_Torque_Mismch) -> Bus Selector1/1, Out2/1  "EngTrqMismchType"
  Bus Selector1/1 -> ECM_CompDiag/3(Eng_Torq_Msmch)  "<Eng_Torque_Mismch_Critical>"
  Override  engTrqCmd/1(Out1) -> ECM_CompDiag/2(engTrqCmdRecvd_SigValid)

== system Clutchless_P2_Parallel_ETE/Clutchless_HSC_ETE/HSC/Camaro Fault Detection/Component Diagnostic/Override Driver Status ==
  note: This subsystem is used to override the model value of a signal to a constant value
  note: Override Switch Subsystem
  In1 : Inport
  Data Type Conversion3 : DataTypeConversion
  Override Value : Constant  OutDataTypeStr=double
  Override_Driver_Status : Constant  Value=0
  Switch : Switch  Criteria=u2 > Threshold
  Out1 : Outport
  wires:
  Override_Driver_Status/1 -> Switch/2
  In1/1 -> Data Type Conversion3/1
  Switch/1 -> Out1/1
  Override Value/1 -> Switch/1
  Data Type Conversion3/1 -> Switch/3

== system Clutchless_P2_Parallel_ETE/Clutchless_HSC_ETE/HSC/Camaro Fault Detection/Component Diagnostic/Override ESS Status ==
  note: This subsystem is used to override the model value of a signal to a constant value
  note: Override Switch Subsystem
  In1 : Inport
  Data Type Conversion3 : DataTypeConversion
  Override Value : Constant  Value=2  OutDataTypeStr=double
  Override_ESS_Status : Constant  Value=0
  Switch : Switch  Criteria=u2 > Threshold
  Terminator : Terminator
  Out1 : Outport
  wires:
  Switch/1 -> Terminator/1
  In1/1 -> Data Type Conversion3/1
  Override_ESS_Status/1 -> Switch/2
  Override Value/1 -> Out1/1, Switch/1
  Data Type Conversion3/1 -> Switch/3

== system Clutchless_P2_Parallel_ETE/Clutchless_HSC_ETE/HSC/Camaro Fault Detection/Component Diagnostic/Override Engine Status ==
  note: This subsystem is used to override the model value of a signal to a constant value
  note: Override Switch Subsystem
  In1 : Inport
  Data Type Conversion3 : DataTypeConversion
  Override Value1 : Constant  Value=2  OutDataTypeStr=double
  Override_Engine_Status : Constant  Value=0
  Switch : Switch  Criteria=u2 > Threshold
  Terminator : Terminator
  Out1 : Outport
  wires:
  Switch/1 -> Terminator/1
  In1/1 -> Data Type Conversion3/1
  Override Value1/1 -> Out1/1, Switch/1
  Override_Engine_Status/1 -> Switch/2
  Data Type Conversion3/1 -> Switch/3

== system Clutchless_P2_Parallel_ETE/Clutchless_HSC_ETE/HSC/Camaro Fault Detection/Component Diagnostic/Override TCM Status ==
  note: This subsystem is used to override the model value of a signal to a constant value
  note: Override Switch Subsystem
  In1 : Inport
  Data Type Conversion3 : DataTypeConversion
  Override Value1 : Constant  Value=2  OutDataTypeStr=double
  Override_TCM_Status : Constant  Value=0
  Switch : Switch  Criteria=u2 > Threshold
  Out1 : Outport
  wires:
  In1/1 -> Data Type Conversion3/1
  Switch/1 -> Out1/1
  Override_TCM_Status/1 -> Switch/2
  Override Value1/1 -> Switch/1
  Data Type Conversion3/1 -> Switch/3

== system Clutchless_P2_Parallel_ETE/Clutchless_HSC_ETE/HSC/Camaro Fault Detection/Component Diagnostic/Transmission Component Diagnostic ==
  In1 : Inport
  Bus Selector : BusSelector  OutputSignals=Transmission_SigDiag.TCMRollingAliveActive_SigValid,Transmission_SigDiag.LvrPosTrnsShft_SigValid,Transmission_SigDiag.TransEstGear_SigValid,Transmission_SigDiag.LockupCmd_SigValid,Transmission_SigDiag.VehDirFault
  TCM_CompDia : Stateflow chart  TreatAsAtomicUnit=on
  Out1 : Outport
  wires:
  In1/1 -> Bus Selector/1
  Bus Selector/1 -> TCM_CompDia/1(TCMRollingAliveActive_SigValid)  "<TCMRollingAliveActive_SigValid>"
  Bus Selector/2 -> TCM_CompDia/2(LvrPosTrnsShft_SigValid)  "<LvrPosTrnsShft_SigValid>"
  Bus Selector/3 -> TCM_CompDia/3(TransEstGear_SigValid)  "<TransEstGear_SigValid>"
  Bus Selector/4 -> TCM_CompDia/4(LockupCmd_SigValid)  "<LockupCmd_SigValid>"
  TCM_CompDia/1(TCM_Status) -> Out1/1  "TCM_Status"
  Bus Selector/5 -> TCM_CompDia/5(VehDirFault)  "<VehDirFault>"

== system Clutchless_P2_Parallel_ETE/Clutchless_HSC_ETE/HSC/Camaro Fault Detection/Input Conversions/BMS_Conversions ==
  note: Fehler_HS_verschweisst
      | 1 : Error: Main contactor welded
  note: BMS_IstModus
      | actual state of the battery / Current status of the battery
      | 0 : Standby ; communication active
      | 1 : main contactors closed / HV power activated / normal driving
      | 2 : closed / Balancing mode main contactors activated
      | 3 : external charging via charger High
      | 4 : external charging HV
      | 5 : Error Battery
      | 6 : External DC Charging HV
      | 7 : Init
  note: MO_BMS_Sollmodus
      | The battery mode is requested:
      | 0: Standby; communication active
      | 1: HV power enable / normal driving mode
      | 2: Balancing Mode
      | 3: HV power enable / external_load_external start
      | 4: HV power enable / external load_EV_PlugIn
      | 5: None
  note: 1 : Error Insulation
  note: 5: error
  note: hvBusVolt_V
  note: hvBattVolt_V
  note: BMS: Conversions and Override Switches
      | (Battery Management System)
  In1 : Inport
  Bus Creator : BusCreator  Inputs=11
  Bus Selector : BusSelector  OutputSignals=from_CAN.fromHV_CAN.from_BMSHybrid.BMS_HYB_02.BMS_HYB_02_BZ,from_CAN.fromHV_CAN.from_BMSHybrid.BMS_HYB_02.BMS_IstModus,from_CAN.fromHV_CAN.from_BMSHybrid.BMS_HYB_02.BMS_IstStrom,from_CAN.fromHV_CAN.from_BMSHybrid.BMS_SOC,from_CAN.fromHV_CAN.from_BMSHybrid.BMS_HYB_02.BMS_IstSpannung,from_CAN.fromHV_CAN.from_BMSHybrid.BMS_Spannung_ZwKr,from_CAN.fromHV_CAN.from_BMSHybrid.BMS_Temperatur,from_CAN.fromHV_CAN.from_BMSHybrid.BMS_Fehler_Isolation,from_CAN.fromHV_CAN.from_BMSHybrid.BMS_HYB_02.BMS_Fehler_HS_offen,from_CAN.fromHV_CAN.from_BMSHybrid.BMS_Fehler_HS_verschweisst
  Conversion  BMS_gdf : DataTypeConversion  OutDataTypeStr=boolean
  Conversion  Fehler_HS_offen : DataTypeConversion  OutDataTypeStr=boolean
  Conversion  Fehler_HS_verschweisst : DataTypeConversion  OutDataTypeStr=boolean
  Conversion  closeContactorsCmd : DataTypeConversion  OutDataTypeStr=boolean
  Conversion  contactorsClsd : DataTypeConversion  OutDataTypeStr=boolean
  Conversion  essTemp_K : DataTypeConversion  OutDataTypeStr=double
  Conversion  hvBattVolt_V : DataTypeConversion  OutDataTypeStr=double
  Conversion  hvBusVolt_V : DataTypeConversion  OutDataTypeStr=double
  Conversion  rollingAliveCnt : DataTypeConversion  OutDataTypeStr=int8
  Conversion essCur_A : DataTypeConversion  OutDataTypeStr=double
  Conversion essSOC_0_1 : DataTypeConversion  OutDataTypeStr=double
  K to C : Bias  Bias=-273.15
  Override  BMS_gdf 0_1 : Subsystem
  Override  closeContactorsCmd : Subsystem
  Override  contactorsClsd : Subsystem
  Override  essCur_A : Subsystem
  Override  essSOC_0_1 : Subsystem
  Override  essTemp_C : Subsystem
  Override  hvBattVolt_V : Subsystem
  Override  hvBusVolt_V : Subsystem
  Override  rollingAliveCnt [1_3] : Subsystem
  Override Fehler_HS_offen : Subsystem
  Override Fehler_HS_verschweisst : Subsystem
  Out1 : Outport
  wires:
  In1/1 -> Bus Selector/1
  Conversion  rollingAliveCnt/1 -> Override  rollingAliveCnt [1_3]/1(In1)
  Override  rollingAliveCnt [1_3]/1(Out1) -> Bus Creator/1  "BMSrollingAliveCnt [123]"
  Bus Creator/1 -> Out1/1  "BMS_Conv"
  Conversion  closeContactorsCmd/1 -> Override  closeContactorsCmd/1(In1)
  Override  closeContactorsCmd/1(Out1) -> Bus Creator/2  "MO_BMS_Sollmodus [0-5]"
  Conversion  contactorsClsd/1 -> Override  contactorsClsd/1(In1)
  Conversion essCur_A/1 -> Override  essCur_A/1(In1)
  Conversion essSOC_0_1/1 -> Override  essSOC_0_1/1(In1)
  Conversion  hvBattVolt_V/1 -> Override  hvBattVolt_V/1(In1)
  Conversion  hvBusVolt_V/1 -> Override  hvBusVolt_V/1(In1)
  Override  contactorsClsd/1(Out1) -> Bus Creator/3  "contactorsClsd"
  Override  essSOC_0_1/1(Out1) -> Bus Creator/5  "essSOC_0_1"
  Override  hvBattVolt_V/1(Out1) -> Bus Creator/6  "hvBattVolt_V"
  Override  essCur_A/1(Out1) -> Bus Creator/4  "essCur_A"
  Override  hvBusVolt_V/1(Out1) -> Bus Creator/7  "hvBusVolt_V"
  Conversion  essTemp_K/1 -> K to C/1
  Override  essTemp_C/1(Out1) -> Bus Creator/8  "essTemp_C"
  K to C/1 -> Override  essTemp_C/1(In1)
  Conversion  BMS_gdf/1 -> Override  BMS_gdf 0_1/1(In1)
  Override  BMS_gdf 0_1/1(Out1) -> Bus Creator/9  "BMS_gdf"
  Bus Selector/2 -> Conversion  contactorsClsd/1  "<BMS_IstModus>"
  Bus Selector/7 -> Conversion  essTemp_K/1  "<BMS_Temperatur>"
  Bus Selector/8 -> Conversion  BMS_gdf/1  "<BMS_Fehler_Isolation>"
  Bus Selector/5 -> Conversion  hvBattVolt_V/1  "<BMS_IstSpannung>"
  Bus Selector/4 -> Conversion essSOC_0_1/1  "<BMS_SOC>"
  Bus Selector/3 -> Conversion essCur_A/1  "<BMS_IstStrom>"
  Bus Selector/1 -> Conversion  rollingAliveCnt/1  "<BMS_HYB_02_BZ>"
  Bus Selector/6 -> Conversion  hvBusVolt_V/1  "<BMS_Spannung_ZwKr>"
  [MO_BMS_Sollmodus] -> Conversion  closeContactorsCmd/1
  Bus Selector/9 -> Conversion  Fehler_HS_offen/1  "<BMS_Fehler_HS_offen>"
  Conversion  Fehler_HS_offen/1 -> Override Fehler_HS_offen/1(In1)
  Override Fehler_HS_offen/1(Out1) -> Bus Creator/10  "Fehler_HS_offen"
  Bus Selector/10 -> Conversion  Fehler_HS_verschweisst/1  "<BMS_Fehler_HS_verschweisst>"
  Conversion  Fehler_HS_verschweisst/1 -> Override Fehler_HS_verschweisst/1(In1)
  Override Fehler_HS_verschweisst/1(Out1) -> Bus Creator/11  "Fehler_HS_verschweisst"

== system Clutchless_P2_Parallel_ETE/Clutchless_HSC_ETE/HSC/Camaro Fault Detection/Input Conversions/DriverInput_Conversions ==
  note: SysPwrMd (EC3)
      | 0 - Off
      | 1 -  Accessory
      | 2 - Run
      | 3 - Crank Request
  note: Driver Controls: Conversions and Override Switches
  In1 : Inport
  Bus Creator : BusCreator  Inputs=7
  Bus Selector : BusSelector  OutputSignals=from_Analog.Driver_APP1,from_Analog.Driver_APP2,from_CAN.fromVEH_CAN.from_BCM.BrkPdlPos,from_CAN.fromVEH_CAN.from_BCM.SysPwrMd,from_CAN.fromVEH_CAN.from_TCM.TrnsShftLvrPos,from_CAN.fromEBCAN.from_ECM.VehSpdAvgDrvn,from_Digital.SW_Regen_Disable
  Conversion  APP1 (%) : DataTypeConversion  OutDataTypeStr=double
  Conversion  APP2 (%) : DataTypeConversion  OutDataTypeStr=double
  Conversion  BPP (%) : DataTypeConversion  OutDataTypeStr=double
  Conversion  KeyPos [0_3] : DataTypeConversion  OutDataTypeStr=int8
  Conversion  V [mph] : DataTypeConversion  OutDataTypeStr=double
  Conversion PRNDL : DataTypeConversion  OutDataTypeStr=uint8
  Conversion Regen : DataTypeConversion  OutDataTypeStr=uint8
  Override  KeyPos [0_3] : Subsystem
  Override APP (%) : Subsystem
  Override APP (%)1 : Subsystem
  Override BPP (%) : Subsystem
  Override PRNDL : Subsystem
  Override Regen : Subsystem
  Override V [mph] : Subsystem
  Out1 : Outport
  wires:
  In1/1 -> Bus Selector/1
  Conversion  APP1 (%)/1 -> Override APP (%)/1(In1)
  Override APP (%)/1(Out1) -> Bus Creator/1  "APP1 [%]"
  Bus Selector/1 -> Conversion  APP1 (%)/1  "<Driver_APP1>"
  Bus Selector/3 -> Conversion  BPP (%)/1  "<BrkPdlPos>"
  Bus Selector/4 -> Conversion  KeyPos [0_3]/1  "<SysPwrMd>"
  Conversion  KeyPos [0_3]/1 -> Override  KeyPos [0_3]/1(In1)
  Override BPP (%)/1(Out1) -> Bus Creator/3  "BPP [%]"
  Override  KeyPos [0_3]/1(Out1) -> Bus Creator/4  "keyPos [0_3]"
  Bus Creator/1 -> Out1/1  "DriverControls_Conv"
  Conversion  BPP (%)/1 -> Override BPP (%)/1(In1)
  Conversion PRNDL/1 -> Override PRNDL/1(In1)
  Override PRNDL/1(Out1) -> Bus Creator/5  "PRNDL"
  Bus Selector/2 -> Conversion  APP2 (%)/1  "<Driver_APP2>"
  Bus Selector/5 -> Conversion PRNDL/1  "<TrnsShftLvrPos>"
  Override APP (%)1/1(Out1) -> Bus Creator/2  "APP2[%]"
  Conversion  APP2 (%)/1 -> Override APP (%)1/1(In1)
  Bus Selector/6 -> Conversion  V [mph]/1  "<VehSpdAvgDrvn>"
  Conversion  V [mph]/1 -> Override V [mph]/1(In1)
  Override V [mph]/1(Out1) -> Bus Creator/6  "V [mph]"
  Bus Selector/7 -> Conversion Regen/1  "<SW_Regen_Disable>"
  Conversion Regen/1 -> Override Regen/1(In1)
  Override Regen/1(Out1) -> Bus Creator/7  "SW_Regen"
